simulink subsystem "sub2"  (R2020a)
settings: Solver=VariableStepAuto  StartTime=0.0  StopTime=10.0  RelTol=1e-3
settings Model: Creator=ecs  LastModifiedBy=ecs

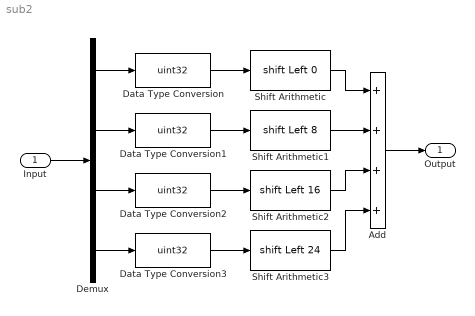
== system sub2 ==
  Input : Inport  OutDataTypeStr=uint8
  Add : Sum  Inputs=++++
  Data Type Conversion{,1..3} (4 alike) : DataTypeConversion  OutDataTypeStr=uint32
  Demux : Demux
  Shift Arithmetic : ArithShift  BitShiftDirection=Left
  Shift Arithmetic1 : ArithShift  BitShiftNumber=8  BitShiftDirection=Left
  Shift Arithmetic2 : ArithShift  BitShiftNumber=16  BitShiftDirection=Left
  Shift Arithmetic3 : ArithShift  BitShiftNumber=24  BitShiftDirection=Left
  Output : Outport
  wires:
  Add/1 -> Output/1
  Shift Arithmetic3/1 -> Add/4
  Data Type Conversion2/1 -> Shift Arithmetic2/1
  Shift Arithmetic2/1 -> Add/3
  Data Type Conversion1/1 -> Shift Arithmetic1/1
  Shift Arithmetic1/1 -> Add/2
  Data Type Conversion/1 -> Shift Arithmetic/1
  Shift Arithmetic/1 -> Add/1
  Data Type Conversion3/1 -> Shift Arithmetic3/1
  Demux/4 -> Data Type Conversion3/1
  Demux/3 -> Data Type Conversion2/1
  Demux/2 -> Data Type Conversion1/1
  Demux/1 -> Data Type Conversion/1
  Input/1 -> Demux/1
